simulink model "ModeStatAndRsp"  (R2018b)
settings: Solver=FixedStepDiscrete  StartTime=0.0  StopTime=10.0  FixedStep=0.01  RelTol=1e-3
undefined symbols (not defined in the file): c_RecvL, c_RecvLR, c_RecvR, IfVeSMSeStNumConfig, KeSMSbMdChime2Enable_Val, KeSMSbSRSPosNumConfig_Val, KeSMSuChmReqDurnTm_Val, KeSMSuChmReqIntlTm_Val, KeSMSuRspStatHldTm_Val, MdRspLocal1, MdTp1, ModeNum, PowerMode1, SrcReqTp1, srsconvert
libraries: RspLib x47, simulink x1
(part 5 of 8)

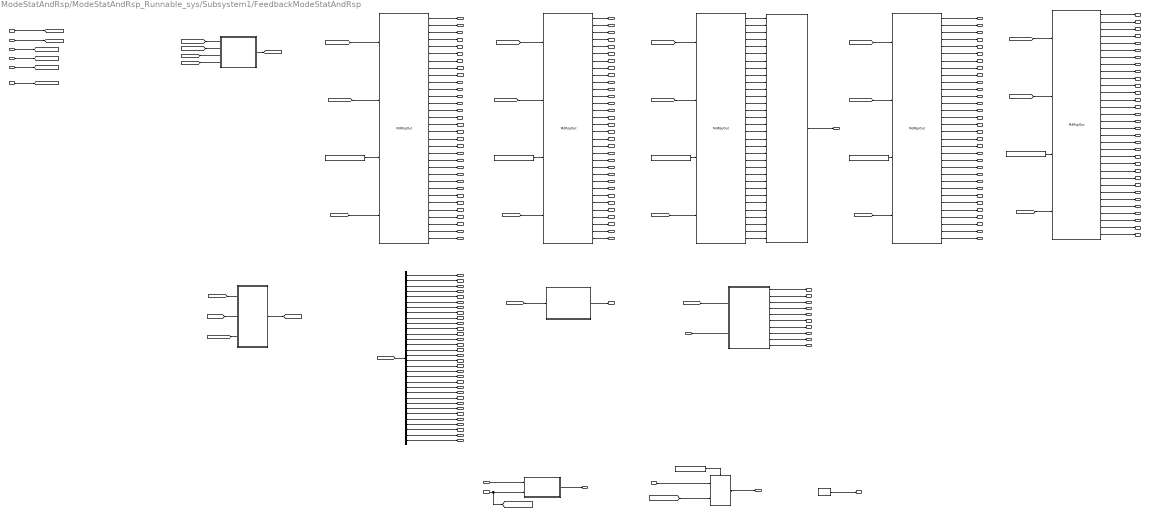
== system ModeStatAndRsp/ModeStatAndRsp_Runnable_sys/Subsystem1/FeedbackModeStatAndRsp ==
  note: REQ_MSM_479
  note: <REQ_MSM_528>
  note: <REQ_MSM_490><REQ_MSM_491>
  note: <REQ_MSM_495>
  note: <REQ_MSM_489>
  note: <REQ_MSM_492><REQ_MSM_493>
  note: <REQ_MSM_492><REQ_MSM_493>
  note: <REQ_MSM_492> <REQ_MSM_493>
  note: 0x3A6
  note: SRSLIN
  note: 0x3A7
  note: <REQ_MSM_270><REQ_MSM_ 405 > <REQ_MSM_ 416 >
  rspStateHldTm : Inport
  PwrMdChked : Inport  Port=2
  ChmMgrStat : Inport  Port=3
  ModeState32 : Inport  Port=4
  ModeStateBus : Inport  Port=5
  isArrivedAtTargetPos : Inport  Port=6
  ModeSrcTp : Inport  Port=7
  ModeRsp : Inport  Port=8
  PosArray_Val_read : Inport  Port=9
  MdExit : Inport  Port=10
  All32in1 : Subsystem
  Bus Selector : BusSelector  OutputSignals=Md1Stat,Md2Stat,Md3Stat,Md4Stat,Md5Stat,Md6Stat,Md7Stat,Md8Stat,Md9Stat,Md10Stat,Md11Stat,Md12Stat,Md13Stat,Md14Stat,Md15Stat,Md16Stat,Md17Stat,Md18Stat,Md19Stat,Md20Stat,Md21Stat,Md22Stat,Md23Stat,Md24Stat,Md25Stat,Md26Stat,Md27Stat,Md28Stat,Md29Stat,Md30Stat,Md31Stat,Md32Stat
  Chime2_3A6 : Subsystem
  Constant : Constant  Value=3  OutDataTypeStr=uint8
  Constant4 : Constant  Value=SrcReqTp1.SrcReqTp_Remote  OutDataTypeStr=Enum:SrcReqTp1
  Constant5 : Constant  Value=SrcReqTp1.SrcReqTp_HMI  OutDataTypeStr=Enum:SrcReqTp1
  Constant6 : Constant  Value=SrcReqTp1.SrcReqTp_SRS  OutDataTypeStr=Enum:SrcReqTp1
  Constant7 : Constant  Value=SrcReqTp1.SrcReqTp_HMI2L  OutDataTypeStr=Enum:SrcReqTp1
  Constant8 : Constant  Value=SrcReqTp1.SrcReqTp_HMI2R  OutDataTypeStr=Enum:SrcReqTp1
  FeedbackPassCmprtHMIDisCmd : Subsystem
  MdRspOut{1..5} (5 alike) : RspLib/MdRspOut  SystemSampleTime=-1
  MdStatComm : Subsystem
  PA_KeSMSbMdChime2Enable_Val : Constant  Value=KeSMSbMdChime2Enable_Val
  RspComm : Subsystem
  StPassCmprtMdCrtMdStat_3A6 : Subsystem
  Subsystem3 : Subsystem
  StPassCmprtMdHMIDisCmd : Outport  VectorParamsAs1DForOutWhenUnconnected=on
  IfVeSMSeStPassCmprtMdNoti2ChmEvntStat_Val_write : Outport  Port=2  VectorParamsAs1DForOutWhenUnconnected=on
  SRSCrtMdIndTyp_67_2_Val_write : Outport  Port=3  VectorParamsAs1DForOutWhenUnconnected=on
  StPassCmprtMdCrtMdStat : Outport  Port=4
  StPassCmprtMd1RclRspStat : Outport  Port=5  VectorParamsAs1DForOutWhenUnconnected=on
  StPassCmprtMd2RclRspStat : Outport  Port=6  VectorParamsAs1DForOutWhenUnconnected=on
  StPassCmprtMd3RclRspStat : Outport  Port=7  VectorParamsAs1DForOutWhenUnconnected=on
  StPassCmprtMd4RclRspStat : Outport  Port=8  VectorParamsAs1DForOutWhenUnconnected=on
  StPassCmprtMd5RclRspStat : Outport  Port=9  VectorParamsAs1DForOutWhenUnconnected=on
  StPassCmprtMd6RclRspStat : Outport  Port=10  VectorParamsAs1DForOutWhenUnconnected=on
  StPassCmprtMd7RclRspStat : Outport  Port=11  VectorParamsAs1DForOutWhenUnconnected=on
  StPassCmprtMd8RclRspStat : Outport  Port=12  VectorParamsAs1DForOutWhenUnconnected=on
  StPassCmprtMd9RclRspStat : Outport  Port=13  VectorParamsAs1DForOutWhenUnconnected=on
  StPassCmprtMd10RclRspStat : Outport  Port=14  VectorParamsAs1DForOutWhenUnconnected=on
  StPassCmprtMd11RclRspStat : Outport  Port=15  VectorParamsAs1DForOutWhenUnconnected=on
  StPassCmprtMd12RclRspStat : Outport  Port=16  VectorParamsAs1DForOutWhenUnconnected=on
  StPassCmprtMd13RclRspStat : Outport  Port=17  VectorParamsAs1DForOutWhenUnconnected=on
  StPassCmprtMd14RclRspStat : Outport  Port=18  VectorParamsAs1DForOutWhenUnconnected=on
  StPassCmprtMd15RclRspStat : Outport  Port=19  VectorParamsAs1DForOutWhenUnconnected=on
  StPassCmprtMd16RclRspStat : Outport  Port=20  VectorParamsAs1DForOutWhenUnconnected=on
  StPassCmprtMd17RclRspStat : Outport  Port=21  VectorParamsAs1DForOutWhenUnconnected=on
  StPassCmprtMd18RclRspStat : Outport  Port=22  VectorParamsAs1DForOutWhenUnconnected=on
  StPassCmprtMd19RclRspStat : Outport  Port=23  VectorParamsAs1DForOutWhenUnconnected=on
  StPassCmprtMd20RclRspStat : Outport  Port=24  VectorParamsAs1DForOutWhenUnconnected=on
  StPassCmprtMd21RclRspStat : Outport  Port=25  VectorParamsAs1DForOutWhenUnconnected=on
  StPassCmprtMd22RclRspStat : Outport  Port=26  VectorParamsAs1DForOutWhenUnconnected=on
  StPassCmprtMd23RclRspStat : Outport  Port=27  VectorParamsAs1DForOutWhenUnconnected=on
  StPassCmprtMd24RclRspStat : Outport  Port=28  VectorParamsAs1DForOutWhenUnconnected=on
  StPassCmprtMd25RclRspStat : Outport  Port=29  VectorParamsAs1DForOutWhenUnconnected=on
  StPassCmprtMd26RclRspStat : Outport  Port=30  VectorParamsAs1DForOutWhenUnconnected=on
  StPassCmprtMd27RclRspStat : Outport  Port=31  VectorParamsAs1DForOutWhenUnconnected=on
  StPassCmprtMd28RclRspStat : Outport  Port=32  VectorParamsAs1DForOutWhenUnconnected=on
  StPassCmprtMd29RclRspStat : Outport  Port=33  VectorParamsAs1DForOutWhenUnconnected=on
  StPassCmprtMd30RclRspStat : Outport  Port=34  VectorParamsAs1DForOutWhenUnconnected=on
  StPassCmprtMd31RclRspStat : Outport  Port=35  VectorParamsAs1DForOutWhenUnconnected=on
  StPassCmprtMd32RclRspStat : Outport  Port=36  VectorParamsAs1DForOutWhenUnconnected=on
  StPassCmprtMd_RfCtrl_Sw_RclRspStat : Outport  Port=37  VectorParamsAs1DForOutWhenUnconnected=on
  StSrv_StMd1_Rsp : Outport  Port=38  VectorParamsAs1DForOutWhenUnconnected=on
  StSrv_StMd2_Rsp : Outport  Port=39  VectorParamsAs1DForOutWhenUnconnected=on
  StSrv_StMd3_Rsp : Outport  Port=40  VectorParamsAs1DForOutWhenUnconnected=on
  StSrv_StMd4_Rsp : Outport  Port=41  VectorParamsAs1DForOutWhenUnconnected=on
  StSrv_StMd5_Rsp : Outport  Port=42  VectorParamsAs1DForOutWhenUnconnected=on
  StSrv_StMd6_Rsp : Outport  Port=43  VectorParamsAs1DForOutWhenUnconnected=on
  StSrv_StMd7_Rsp : Outport  Port=44  VectorParamsAs1DForOutWhenUnconnected=on
  StSrv_StMd8_Rsp : Outport  Port=45  VectorParamsAs1DForOutWhenUnconnected=on
  StSrv_StMd9_Rsp : Outport  Port=46  VectorParamsAs1DForOutWhenUnconnected=on
  StSrv_StMd10_Rsp : Outport  Port=47  VectorParamsAs1DForOutWhenUnconnected=on
  StSrv_StMd11_Rsp : Outport  Port=48  VectorParamsAs1DForOutWhenUnconnected=on
  StSrv_StMd12_Rsp : Outport  Port=49  VectorParamsAs1DForOutWhenUnconnected=on
  StSrv_StMd13_Rsp : Outport  Port=50  VectorParamsAs1DForOutWhenUnconnected=on
  StSrv_StMd14_Rsp : Outport  Port=51  VectorParamsAs1DForOutWhenUnconnected=on
  StSrv_StMd15_Rsp : Outport  Port=52  VectorParamsAs1DForOutWhenUnconnected=on
  StSrv_StMd16_Rsp : Outport  Port=53  VectorParamsAs1DForOutWhenUnconnected=on
  StSrv_StMd17_Rsp : Outport  Port=54  VectorParamsAs1DForOutWhenUnconnected=on
  StSrv_StMd18_Rsp : Outport  Port=55  VectorParamsAs1DForOutWhenUnconnected=on
  StSrv_StMd19_Rsp : Outport  Port=56  VectorParamsAs1DForOutWhenUnconnected=on
  StSrv_StMd20_Rsp : Outport  Port=57  VectorParamsAs1DForOutWhenUnconnected=on
  StSrv_StMd21_Rsp : Outport  Port=58  VectorParamsAs1DForOutWhenUnconnected=on
  StSrv_StMd22_Rsp : Outport  Port=59  VectorParamsAs1DForOutWhenUnconnected=on
  StSrv_StMd23_Rsp : Outport  Port=60  VectorParamsAs1DForOutWhenUnconnected=on
  StSrv_StMd24_Rsp : Outport  Port=61  VectorParamsAs1DForOutWhenUnconnected=on
  StSrv_StMd25_Rsp : Outport  Port=62  VectorParamsAs1DForOutWhenUnconnected=on
  StSrv_StMd26_Rsp : Outport  Port=63  VectorParamsAs1DForOutWhenUnconnected=on
  StSrv_StMd27_Rsp : Outport  Port=64  VectorParamsAs1DForOutWhenUnconnected=on
  StSrv_StMd28_Rsp : Outport  Port=65  VectorParamsAs1DForOutWhenUnconnected=on
  StSrv_StMd29_Rsp : Outport  Port=66  VectorParamsAs1DForOutWhenUnconnected=on
  StSrv_StMd30_Rsp : Outport  Port=67  VectorParamsAs1DForOutWhenUnconnected=on
  StSrv_StMd31_Rsp : Outport  Port=68  VectorParamsAs1DForOutWhenUnconnected=on
  StSrv_StMd32_Rsp : Outport  Port=69  VectorParamsAs1DForOutWhenUnconnected=on
  HMI_2L_StMd1_Rsp : Outport  Port=70  VectorParamsAs1DForOutWhenUnconnected=on
  HMI_2L_StMd2_Rsp : Outport  Port=71  VectorParamsAs1DForOutWhenUnconnected=on
  HMI_2L_StMd3_Rsp : Outport  Port=72  VectorParamsAs1DForOutWhenUnconnected=on
  HMI_2L_StMd4_Rsp : Outport  Port=73  VectorParamsAs1DForOutWhenUnconnected=on
  HMI_2L_StMd5_Rsp : Outport  Port=74  VectorParamsAs1DForOutWhenUnconnected=on
  HMI_2L_StMd6_Rsp : Outport  Port=75  VectorParamsAs1DForOutWhenUnconnected=on
  HMI_2L_StMd7_Rsp : Outport  Port=76  VectorParamsAs1DForOutWhenUnconnected=on
  HMI_2L_StMd8_Rsp : Outport  Port=77  VectorParamsAs1DForOutWhenUnconnected=on
  HMI_2L_StMd9_Rsp : Outport  Port=78  VectorParamsAs1DForOutWhenUnconnected=on
  HMI_2L_StMd10_Rsp : Outport  Port=79  VectorParamsAs1DForOutWhenUnconnected=on
  HMI_2L_StMd11_Rsp : Outport  Port=80  VectorParamsAs1DForOutWhenUnconnected=on
  HMI_2L_StMd12_Rsp : Outport  Port=81  VectorParamsAs1DForOutWhenUnconnected=on
  HMI_2L_StMd13_Rsp : Outport  Port=82  VectorParamsAs1DForOutWhenUnconnected=on
  HMI_2L_StMd14_Rsp : Outport  Port=83  VectorParamsAs1DForOutWhenUnconnected=on
  HMI_2L_StMd15_Rsp : Outport  Port=84  VectorParamsAs1DForOutWhenUnconnected=on
  HMI_2L_StMd16_Rsp : Outport  Port=85  VectorParamsAs1DForOutWhenUnconnected=on
  HMI_2L_StMd17_Rsp : Outport  Port=86  VectorParamsAs1DForOutWhenUnconnected=on
  HMI_2L_StMd18_Rsp : Outport  Port=87  VectorParamsAs1DForOutWhenUnconnected=on
  HMI_2L_StMd19_Rsp : Outport  Port=88  VectorParamsAs1DForOutWhenUnconnected=on
  HMI_2L_StMd20_Rsp : Outport  Port=89  VectorParamsAs1DForOutWhenUnconnected=on
  HMI_2L_StMd21_Rsp : Outport  Port=90  VectorParamsAs1DForOutWhenUnconnected=on
  HMI_2L_StMd22_Rsp : Outport  Port=91  VectorParamsAs1DForOutWhenUnconnected=on
  HMI_2L_StMd23_Rsp : Outport  Port=92  VectorParamsAs1DForOutWhenUnconnected=on
  HMI_2L_StMd24_Rsp : Outport  Port=93  VectorParamsAs1DForOutWhenUnconnected=on
  HMI_2L_StMd25_Rsp : Outport  Port=94  VectorParamsAs1DForOutWhenUnconnected=on
  HMI_2L_StMd26_Rsp : Outport  Port=95  VectorParamsAs1DForOutWhenUnconnected=on
  HMI_2L_StMd27_Rsp : Outport  Port=96  VectorParamsAs1DForOutWhenUnconnected=on
  HMI_2L_StMd28_Rsp : Outport  Port=97  VectorParamsAs1DForOutWhenUnconnected=on
  HMI_2L_StMd29_Rsp : Outport  Port=98  VectorParamsAs1DForOutWhenUnconnected=on
  HMI_2L_StMd30_Rsp : Outport  Port=99  VectorParamsAs1DForOutWhenUnconnected=on
  HMI_2L_StMd31_Rsp : Outport  Port=100  VectorParamsAs1DForOutWhenUnconnected=on
  HMI_2L_StMd32_Rsp : Outport  Port=101  VectorParamsAs1DForOutWhenUnconnected=on
  HMI_2R_StMd1_Rsp : Outport  Port=102  VectorParamsAs1DForOutWhenUnconnected=on
  HMI_2R_StMd2_Rsp : Outport  Port=103  VectorParamsAs1DForOutWhenUnconnected=on
  HMI_2R_StMd3_Rsp : Outport  Port=104  VectorParamsAs1DForOutWhenUnconnected=on
  HMI_2R_StMd4_Rsp : Outport  Port=105  VectorParamsAs1DForOutWhenUnconnected=on
  HMI_2R_StMd5_Rsp : Outport  Port=106  VectorParamsAs1DForOutWhenUnconnected=on
  HMI_2R_StMd6_Rsp : Outport  Port=107  VectorParamsAs1DForOutWhenUnconnected=on
  HMI_2R_StMd7_Rsp : Outport  Port=108  VectorParamsAs1DForOutWhenUnconnected=on
  HMI_2R_StMd8_Rsp : Outport  Port=109  VectorParamsAs1DForOutWhenUnconnected=on
  HMI_2R_StMd9_Rsp : Outport  Port=110  VectorParamsAs1DForOutWhenUnconnected=on
  HMI_2R_StMd10_Rsp : Outport  Port=111  VectorParamsAs1DForOutWhenUnconnected=on
  HMI_2R_StMd11_Rsp : Outport  Port=112  VectorParamsAs1DForOutWhenUnconnected=on
  HMI_2R_StMd12_Rsp : Outport  Port=113  VectorParamsAs1DForOutWhenUnconnected=on
  HMI_2R_StMd13_Rsp : Outport  Port=114  VectorParamsAs1DForOutWhenUnconnected=on
  HMI_2R_StMd14_Rsp : Outport  Port=115  VectorParamsAs1DForOutWhenUnconnected=on
  HMI_2R_StMd15_Rsp : Outport  Port=116  VectorParamsAs1DForOutWhenUnconnected=on
  HMI_2R_StMd16_Rsp : Outport  Port=117  VectorParamsAs1DForOutWhenUnconnected=on
  HMI_2R_StMd17_Rsp : Outport  Port=118  VectorParamsAs1DForOutWhenUnconnected=on
  HMI_2R_StMd18_Rsp : Outport  Port=119  VectorParamsAs1DForOutWhenUnconnected=on
  HMI_2R_StMd19_Rsp : Outport  Port=120  VectorParamsAs1DForOutWhenUnconnected=on
  HMI_2R_StMd20_Rsp : Outport  Port=121  VectorParamsAs1DForOutWhenUnconnected=on
  HMI_2R_StMd21_Rsp : Outport  Port=122  VectorParamsAs1DForOutWhenUnconnected=on
  HMI_2R_StMd22_Rsp : Outport  Port=123  VectorParamsAs1DForOutWhenUnconnected=on
  HMI_2R_StMd23_Rsp : Outport  Port=124  VectorParamsAs1DForOutWhenUnconnected=on
  HMI_2R_StMd24_Rsp : Outport  Port=125  VectorParamsAs1DForOutWhenUnconnected=on
  HMI_2R_StMd25_Rsp : Outport  Port=126  VectorParamsAs1DForOutWhenUnconnected=on
  HMI_2R_StMd26_Rsp : Outport  Port=127  VectorParamsAs1DForOutWhenUnconnected=on
  HMI_2R_StMd27_Rsp : Outport  Port=128  VectorParamsAs1DForOutWhenUnconnected=on
  HMI_2R_StMd28_Rsp : Outport  Port=129  VectorParamsAs1DForOutWhenUnconnected=on
  HMI_2R_StMd29_Rsp : Outport  Port=130  VectorParamsAs1DForOutWhenUnconnected=on
  HMI_2R_StMd30_Rsp : Outport  Port=131  VectorParamsAs1DForOutWhenUnconnected=on
  HMI_2R_StMd31_Rsp : Outport  Port=132  VectorParamsAs1DForOutWhenUnconnected=on
  HMI_2R_StMd32_Rsp : Outport  Port=133  VectorParamsAs1DForOutWhenUnconnected=on
  StPassCmprtMd_Md1_CrtStat : Outport  Port=134
  StPassCmprtMd_Md2_CrtStat : Outport  Port=135
  StPassCmprtMd_Md3_CrtStat : Outport  Port=136
  StPassCmprtMd_Md4_CrtStat : Outport  Port=137
  StPassCmprtMd_Md5_CrtStat : Outport  Port=138
  StPassCmprtMd_Md6_CrtStat : Outport  Port=139
  StPassCmprtMd_Md7_CrtStat : Outport  Port=140
  StPassCmprtMd_Md8_CrtStat : Outport  Port=141
  StPassCmprtMd_Md9_CrtStat : Outport  Port=142
  StPassCmprtMd_Md10_CrtStat : Outport  Port=143
  StPassCmprtMd_Md11_CrtStat : Outport  Port=144
  StPassCmprtMd_Md12_CrtStat : Outport  Port=145
  StPassCmprtMd_Md13_CrtStat : Outport  Port=146
  StPassCmprtMd_Md14_CrtStat : Outport  Port=147
  StPassCmprtMd_Md15_CrtStat : Outport  Port=148
  StPassCmprtMd_Md16_CrtStat : Outport  Port=149
  StPassCmprtMd_Md17_CrtStat : Outport  Port=150
  StPassCmprtMd_Md18_CrtStat : Outport  Port=151
  StPassCmprtMd_Md19_CrtStat : Outport  Port=152
  StPassCmprtMd_Md20_CrtStat : Outport  Port=153
  StPassCmprtMd_Md21_CrtStat : Outport  Port=154
  StPassCmprtMd_Md22_CrtStat : Outport  Port=155
  StPassCmprtMd_Md23_CrtStat : Outport  Port=156
  StPassCmprtMd_Md24_CrtStat : Outport  Port=157
  StPassCmprtMd_Md25_CrtStat : Outport  Port=158
  StPassCmprtMd_Md26_CrtStat : Outport  Port=159
  StPassCmprtMd_Md27_CrtStat : Outport  Port=160
  StPassCmprtMd_Md28_CrtStat : Outport  Port=161
  StPassCmprtMd_Md29_CrtStat : Outport  Port=162
  StPassCmprtMd_Md30_CrtStat : Outport  Port=163
  StPassCmprtMd_Md31_CrtStat : Outport  Port=164
  StPassCmprtMd_Md32_CrtStat : Outport  Port=165
  SRSCrt_MdSw1_Stat_67_2 : Outport  Port=166
  SRSCrt_MdSw2_Stat_67_2 : Outport  Port=167
  SRSCrt_MdSw3_Stat_67_2 : Outport  Port=168
  SRSCrt_MdSw4_Stat_67_2 : Outport  Port=169
  SRSCrt_MdSw5_Stat_67_2 : Outport  Port=170
  SRSCrt_MdSw6_Stat_67_2 : Outport  Port=171
  SRSCrt_MdSw7_Stat_67_2 : Outport  Port=172
  SRSCrt_MdSw8_Stat_67_2 : Outport  Port=173
  SRSCrt_MdSw9_Stat_67_2 : Outport  Port=174
  SRSCrt_MdSw10_Stat_67_2 : Outport  Port=175
  wires:
  rspStateHldTm/1 -> [rspStateHldTm]
  MdRspOut5/1 -> StPassCmprtMd1RclRspStat/1
  StPassCmprtMdCrtMdStat_3A6/1(StPassCmprtMdCrtMdStat) -> StPassCmprtMdCrtMdStat/1
  FeedbackPassCmprtHMIDisCmd/1(StPassCmprtMdHMIDisCmd) -> StPassCmprtMdHMIDisCmd/1
  PwrMdChked/1 -> FeedbackPassCmprtHMIDisCmd/1(powerMode)
  MdRspOut2/6 -> StSrv_StMd6_Rsp/1
  MdRspOut2/7 -> StSrv_StMd7_Rsp/1
  MdRspOut2/8 -> StSrv_StMd8_Rsp/1
  MdRspOut2/4 -> StSrv_StMd4_Rsp/1
  MdRspOut2/5 -> StSrv_StMd5_Rsp/1
  MdRspOut2/1 -> StSrv_StMd1_Rsp/1
  MdRspOut2/2 -> StSrv_StMd2_Rsp/1
  MdRspOut2/3 -> StSrv_StMd3_Rsp/1
  Constant4/1 -> MdRspOut2/3
  Chime2_3A6/1(Out1) -> IfVeSMSeStPassCmprtMdNoti2ChmEvntStat_Val_write/1
  ChmMgrStat/1 -> Chime2_3A6/1(ChmMgrStat)
  Constant/1 -> SRSCrtMdIndTyp_67_2_Val_write/1
  ModeSrcTp/1 -> [ModeSrcTp]
  ModeRsp/1 -> [ModeRsp]
  ModeStateBus/1 -> [ModeStateBus]
  [MdRsp] -> MdRspOut2/1
  [ModeSrcTp] -> MdRspOut2/2
  [ModeSrcTp] -> MdRspOut5/2
  [MdRsp] -> MdRspOut5/1
  ModeState32/1 -> [ModeState32], FeedbackPassCmprtHMIDisCmd/2(ModeState32)
  [ModeState32] -> Chime2_3A6/2(ModeState32)
  [ModeStateBus] -> RspComm/1(oModeStateBus)
  [ModeRsp] -> RspComm/2(oModeRsp)
  [rspStateHldTm] -> RspComm/3(rspStateHldTm)
  RspComm/1(Rsp) -> [MdRsp]
  MdRspOut5/3 -> StPassCmprtMd3RclRspStat/1
  MdRspOut5/4 -> StPassCmprtMd4RclRspStat/1
  MdRspOut5/2 -> StPassCmprtMd2RclRspStat/1
  MdRspOut5/5 -> StPassCmprtMd5RclRspStat/1
  MdRspOut5/6 -> StPassCmprtMd6RclRspStat/1
  MdRspOut5/7 -> StPassCmprtMd7RclRspStat/1
  MdRspOut5/8 -> StPassCmprtMd8RclRspStat/1
  MdRspOut5/9 -> StPassCmprtMd9RclRspStat/1
  MdRspOut5/10 -> StPassCmprtMd10RclRspStat/1
  MdRspOut5/11 -> StPassCmprtMd11RclRspStat/1
  MdRspOut5/12 -> StPassCmprtMd12RclRspStat/1
  MdRspOut5/13 -> StPassCmprtMd13RclRspStat/1
  MdRspOut5/14 -> StPassCmprtMd14RclRspStat/1
  MdRspOut5/15 -> StPassCmprtMd15RclRspStat/1
  MdRspOut5/16 -> StPassCmprtMd16RclRspStat/1
  MdRspOut5/17 -> StPassCmprtMd17RclRspStat/1
  MdRspOut5/18 -> StPassCmprtMd18RclRspStat/1
  MdRspOut5/19 -> StPassCmprtMd19RclRspStat/1
  MdRspOut5/20 -> StPassCmprtMd20RclRspStat/1
  MdRspOut5/21 -> StPassCmprtMd21RclRspStat/1
  MdRspOut5/22 -> StPassCmprtMd22RclRspStat/1
  MdRspOut5/23 -> StPassCmprtMd23RclRspStat/1
  MdRspOut5/24 -> StPassCmprtMd24RclRspStat/1
  MdRspOut5/25 -> StPassCmprtMd25RclRspStat/1
  MdRspOut5/26 -> StPassCmprtMd26RclRspStat/1
  MdRspOut5/27 -> StPassCmprtMd27RclRspStat/1
  MdRspOut5/28 -> StPassCmprtMd28RclRspStat/1
  MdRspOut5/29 -> StPassCmprtMd29RclRspStat/1
  MdRspOut5/30 -> StPassCmprtMd30RclRspStat/1
  MdRspOut5/31 -> StPassCmprtMd31RclRspStat/1
  MdRspOut5/32 -> StPassCmprtMd32RclRspStat/1
  Constant5/1 -> MdRspOut5/3
  isArrivedAtTargetPos/1 -> [isArrivedAtTargetPos]
  [isArrivedAtTargetPos] -> RspComm/4(IsArrivedAtTrgtPos)
  [MdRsp] -> MdRspOut1/1
  [ModeSrcTp] -> MdRspOut1/2
  Constant6/1 -> MdRspOut1/3
  All32in1/1(Allin1Rsp) -> StPassCmprtMd_RfCtrl_Sw_RclRspStat/1
  MdRspOut1/1 -> All32in1/1(Md1Rsp)
  MdRspOut1/2 -> All32in1/2(Md2Rsp)
  MdRspOut1/3 -> All32in1/3(Md3Rsp)
  MdRspOut1/4 -> All32in1/4(Md4Rsp)
  MdRspOut1/5 -> All32in1/5(Md5Rsp)
  MdRspOut1/6 -> All32in1/6(Md6Rsp)
  MdRspOut1/7 -> All32in1/7(Md7Rsp)
  MdRspOut1/8 -> All32in1/8(Md8Rsp)
  MdRspOut1/9 -> All32in1/9(Md9Rsp)
  MdRspOut1/10 -> All32in1/10(Md10Rsp)
  MdRspOut1/11 -> All32in1/11(Md11Rsp)
  MdRspOut1/12 -> All32in1/12(Md12Rsp)
  MdRspOut1/13 -> All32in1/13(Md13Rsp)
  MdRspOut1/14 -> All32in1/14(Md14Rsp)
  MdRspOut1/15 -> All32in1/15(Md15Rsp)
  MdRspOut1/16 -> All32in1/16(Md16Rsp)
  MdRspOut1/17 -> All32in1/17(Md17Rsp)
  MdRspOut1/18 -> All32in1/18(Md18Rsp)
  MdRspOut1/19 -> All32in1/19(Md19Rsp)
  MdRspOut1/20 -> All32in1/20(Md20Rsp)
  MdRspOut1/21 -> All32in1/21(Md21Rsp)
  MdRspOut1/22 -> All32in1/22(Md22Rsp)
  MdRspOut1/23 -> All32in1/23(Md23Rsp)
  MdRspOut1/24 -> All32in1/24(Md24Rsp)
  MdRspOut1/25 -> All32in1/25(Md25Rsp)
  MdRspOut1/26 -> All32in1/26(Md26Rsp)
  MdRspOut1/27 -> All32in1/27(Md27Rsp)
  MdRspOut1/28 -> All32in1/28(Md28Rsp)
  MdRspOut1/29 -> All32in1/29(Md29Rsp)
  MdRspOut1/30 -> All32in1/30(Md30Rsp)
  MdRspOut1/31 -> All32in1/31(Md31Rsp)
  MdRspOut1/32 -> All32in1/32(Md32Rsp)
  MdRspOut2/9 -> StSrv_StMd9_Rsp/1
  MdRspOut2/10 -> StSrv_StMd10_Rsp/1
  MdRspOut2/11 -> StSrv_StMd11_Rsp/1
  MdRspOut2/12 -> StSrv_StMd12_Rsp/1
  MdRspOut2/13 -> StSrv_StMd13_Rsp/1
  MdRspOut2/14 -> StSrv_StMd14_Rsp/1
  MdRspOut2/15 -> StSrv_StMd15_Rsp/1
  MdRspOut2/16 -> StSrv_StMd16_Rsp/1
  MdRspOut2/17 -> StSrv_StMd17_Rsp/1
  MdRspOut2/18 -> StSrv_StMd18_Rsp/1
  MdRspOut2/19 -> StSrv_StMd19_Rsp/1
  MdRspOut2/20 -> StSrv_StMd20_Rsp/1
  MdRspOut2/21 -> StSrv_StMd21_Rsp/1
  MdRspOut2/22 -> StSrv_StMd22_Rsp/1
  MdRspOut2/23 -> StSrv_StMd23_Rsp/1
  MdRspOut2/24 -> StSrv_StMd24_Rsp/1
  MdRspOut2/25 -> StSrv_StMd25_Rsp/1
  MdRspOut2/26 -> StSrv_StMd26_Rsp/1
  MdRspOut2/27 -> StSrv_StMd27_Rsp/1
  MdRspOut2/28 -> StSrv_StMd28_Rsp/1
  MdRspOut2/29 -> StSrv_StMd29_Rsp/1
  MdRspOut2/30 -> StSrv_StMd30_Rsp/1
  MdRspOut2/31 -> StSrv_StMd31_Rsp/1
  MdRspOut2/32 -> StSrv_StMd32_Rsp/1
  [MdRsp] -> MdRspOut3/1
  [ModeSrcTp] -> MdRspOut3/2
  Constant7/1 -> MdRspOut3/3
  [ModeSrcTp] -> MdRspOut4/2
  [MdRsp] -> MdRspOut4/1
  Constant8/1 -> MdRspOut4/3
  MdRspOut3/1 -> HMI_2L_StMd1_Rsp/1
  MdRspOut3/2 -> HMI_2L_StMd2_Rsp/1
  MdRspOut3/3 -> HMI_2L_StMd3_Rsp/1
  MdRspOut3/4 -> HMI_2L_StMd4_Rsp/1
  MdRspOut3/5 -> HMI_2L_StMd5_Rsp/1
  MdRspOut3/6 -> HMI_2L_StMd6_Rsp/1
  MdRspOut3/7 -> HMI_2L_StMd7_Rsp/1
  MdRspOut3/8 -> HMI_2L_StMd8_Rsp/1
  MdRspOut3/9 -> HMI_2L_StMd9_Rsp/1
  MdRspOut3/10 -> HMI_2L_StMd10_Rsp/1
  MdRspOut3/11 -> HMI_2L_StMd11_Rsp/1
  MdRspOut3/12 -> HMI_2L_StMd12_Rsp/1
  MdRspOut3/13 -> HMI_2L_StMd13_Rsp/1
  MdRspOut3/14 -> HMI_2L_StMd14_Rsp/1
  MdRspOut3/15 -> HMI_2L_StMd15_Rsp/1
  MdRspOut3/16 -> HMI_2L_StMd16_Rsp/1
  MdRspOut3/17 -> HMI_2L_StMd17_Rsp/1
  MdRspOut3/18 -> HMI_2L_StMd18_Rsp/1
  MdRspOut3/19 -> HMI_2L_StMd19_Rsp/1
  MdRspOut3/20 -> HMI_2L_StMd20_Rsp/1
  MdRspOut3/21 -> HMI_2L_StMd21_Rsp/1
  MdRspOut3/22 -> HMI_2L_StMd22_Rsp/1
  MdRspOut3/23 -> HMI_2L_StMd23_Rsp/1
  MdRspOut3/24 -> HMI_2L_StMd24_Rsp/1
  MdRspOut3/25 -> HMI_2L_StMd25_Rsp/1
  MdRspOut3/26 -> HMI_2L_StMd26_Rsp/1
  MdRspOut3/27 -> HMI_2L_StMd27_Rsp/1
  MdRspOut3/28 -> HMI_2L_StMd28_Rsp/1
  MdRspOut3/29 -> HMI_2L_StMd29_Rsp/1
  MdRspOut3/30 -> HMI_2L_StMd30_Rsp/1
  MdRspOut3/31 -> HMI_2L_StMd31_Rsp/1
  MdRspOut3/32 -> HMI_2L_StMd32_Rsp/1
  MdRspOut4/1 -> HMI_2R_StMd1_Rsp/1
  MdRspOut4/31 -> HMI_2R_StMd31_Rsp/1
  MdRspOut4/29 -> HMI_2R_StMd29_Rsp/1
  MdRspOut4/28 -> HMI_2R_StMd28_Rsp/1
  MdRspOut4/26 -> HMI_2R_StMd26_Rsp/1
  MdRspOut4/32 -> HMI_2R_StMd32_Rsp/1
  MdRspOut4/27 -> HMI_2R_StMd27_Rsp/1
  MdRspOut4/23 -> HMI_2R_StMd23_Rsp/1
  MdRspOut4/24 -> HMI_2R_StMd24_Rsp/1
  MdRspOut4/22 -> HMI_2R_StMd22_Rsp/1
  MdRspOut4/19 -> HMI_2R_StMd19_Rsp/1
  MdRspOut4/20 -> HMI_2R_StMd20_Rsp/1
  MdRspOut4/18 -> HMI_2R_StMd18_Rsp/1
  MdRspOut4/16 -> HMI_2R_StMd16_Rsp/1
  MdRspOut4/17 -> HMI_2R_StMd17_Rsp/1
  MdRspOut4/15 -> HMI_2R_StMd15_Rsp/1
  MdRspOut4/12 -> HMI_2R_StMd12_Rsp/1
  MdRspOut4/11 -> HMI_2R_StMd11_Rsp/1
  MdRspOut4/10 -> HMI_2R_StMd10_Rsp/1
  MdRspOut4/5 -> HMI_2R_StMd5_Rsp/1
  MdRspOut4/7 -> HMI_2R_StMd7_Rsp/1
  MdRspOut4/30 -> HMI_2R_StMd30_Rsp/1
  MdRspOut4/8 -> HMI_2R_StMd8_Rsp/1
  MdRspOut4/21 -> HMI_2R_StMd21_Rsp/1
  MdRspOut4/6 -> HMI_2R_StMd6_Rsp/1
  MdRspOut4/4 -> HMI_2R_StMd4_Rsp/1
  MdRspOut4/25 -> HMI_2R_StMd25_Rsp/1
  MdRspOut4/3 -> HMI_2R_StMd3_Rsp/1
  MdRspOut4/13 -> HMI_2R_StMd13_Rsp/1
  MdRspOut4/2 -> HMI_2R_StMd2_Rsp/1
  MdRspOut4/9 -> HMI_2R_StMd9_Rsp/1
  MdRspOut4/14 -> HMI_2R_StMd14_Rsp/1
  [isArrivedAtTargetPos] -> MdStatComm/1(IsArrivedAtTrgtPos)
  [MdRsp] -> MdStatComm/2(Rsp)
  MdStatComm/1(MdStat) -> [MdStat]
  [MdStat] -> Bus Selector/1
  Bus Selector/1 -> StPassCmprtMd_Md1_CrtStat/1  "<Md1Stat>"
  Bus Selector/2 -> StPassCmprtMd_Md2_CrtStat/1  "<Md2Stat>"
  Bus Selector/3 -> StPassCmprtMd_Md3_CrtStat/1  "<Md3Stat>"
  Bus Selector/4 -> StPassCmprtMd_Md4_CrtStat/1  "<Md4Stat>"
  Bus Selector/5 -> StPassCmprtMd_Md5_CrtStat/1  "<Md5Stat>"
  Bus Selector/6 -> StPassCmprtMd_Md6_CrtStat/1  "<Md6Stat>"
  Bus Selector/7 -> StPassCmprtMd_Md7_CrtStat/1  "<Md7Stat>"
  Bus Selector/8 -> StPassCmprtMd_Md8_CrtStat/1  "<Md8Stat>"
  Bus Selector/9 -> StPassCmprtMd_Md9_CrtStat/1  "<Md9Stat>"
  Bus Selector/10 -> StPassCmprtMd_Md10_CrtStat/1  "<Md10Stat>"
  Bus Selector/11 -> StPassCmprtMd_Md11_CrtStat/1  "<Md11Stat>"
  Bus Selector/12 -> StPassCmprtMd_Md12_CrtStat/1  "<Md12Stat>"
  Bus Selector/13 -> StPassCmprtMd_Md13_CrtStat/1  "<Md13Stat>"
  Bus Selector/14 -> StPassCmprtMd_Md14_CrtStat/1  "<Md14Stat>"
  Bus Selector/15 -> StPassCmprtMd_Md15_CrtStat/1  "<Md15Stat>"
  Bus Selector/16 -> StPassCmprtMd_Md16_CrtStat/1  "<Md16Stat>"
  Bus Selector/17 -> StPassCmprtMd_Md17_CrtStat/1  "<Md17Stat>"
  Bus Selector/18 -> StPassCmprtMd_Md18_CrtStat/1  "<Md18Stat>"
  Bus Selector/19 -> StPassCmprtMd_Md19_CrtStat/1  "<Md19Stat>"
  Bus Selector/20 -> StPassCmprtMd_Md20_CrtStat/1  "<Md20Stat>"
  Bus Selector/21 -> StPassCmprtMd_Md21_CrtStat/1  "<Md21Stat>"
  Bus Selector/22 -> StPassCmprtMd_Md22_CrtStat/1  "<Md22Stat>"
  Bus Selector/23 -> StPassCmprtMd_Md23_CrtStat/1  "<Md23Stat>"
  Bus Selector/24 -> StPassCmprtMd_Md24_CrtStat/1  "<Md24Stat>"
  Bus Selector/25 -> StPassCmprtMd_Md25_CrtStat/1  "<Md25Stat>"
  Bus Selector/26 -> StPassCmprtMd_Md26_CrtStat/1  "<Md26Stat>"
  Bus Selector/27 -> StPassCmprtMd_Md27_CrtStat/1  "<Md27Stat>"
  Bus Selector/28 -> StPassCmprtMd_Md28_CrtStat/1  "<Md28Stat>"
  Bus Selector/29 -> StPassCmprtMd_Md29_CrtStat/1  "<Md29Stat>"
  Bus Selector/30 -> StPassCmprtMd_Md30_CrtStat/1  "<Md30Stat>"
  Bus Selector/31 -> StPassCmprtMd_Md31_CrtStat/1  "<Md31Stat>"
  Bus Selector/32 -> StPassCmprtMd_Md32_CrtStat/1  "<Md32Stat>"
  [MdStat] -> StPassCmprtMdCrtMdStat_3A6/1(MdStat)
  Subsystem3/9(SRSCrt_MdSw9_Stat_67_2) -> SRSCrt_MdSw9_Stat_67_2/1
  Subsystem3/5(SRSCrt_MdSw5_Stat_67_2) -> SRSCrt_MdSw5_Stat_67_2/1
  Subsystem3/6(SRSCrt_MdSw6_Stat_67_2) -> SRSCrt_MdSw6_Stat_67_2/1
  Subsystem3/7(SRSCrt_MdSw7_Stat_67_2) -> SRSCrt_MdSw7_Stat_67_2/1
  Subsystem3/8(SRSCrt_MdSw8_Stat_67_2) -> SRSCrt_MdSw8_Stat_67_2/1
  Subsystem3/3(SRSCrt_MdSw3_Stat_67_2) -> SRSCrt_MdSw3_Stat_67_2/1
  Subsystem3/4(SRSCrt_MdSw4_Stat_67_2) -> SRSCrt_MdSw4_Stat_67_2/1
  Subsystem3/10(SRSCrt_MdSw10_Stat_67_2) -> SRSCrt_MdSw10_Stat_67_2/1
  Subsystem3/1(SRSCrt_MdSw1_Stat_67_2) -> SRSCrt_MdSw1_Stat_67_2/1
  Subsystem3/2(SRSCrt_MdSw2_Stat_67_2) -> SRSCrt_MdSw2_Stat_67_2/1
  [MdStat] -> Subsystem3/1(MdStat)
  PosArray_Val_read/1 -> Subsystem3/2(PosArray_Val_read)
  [rspStateHldTm] -> MdRspOut2/4
  [rspStateHldTm] -> MdRspOut5/4
  [rspStateHldTm] -> MdRspOut1/4
  [rspStateHldTm] -> MdRspOut3/4
  [rspStateHldTm] -> MdRspOut4/4
  MdExit/1 -> [MdExit]
  [MdExit] -> MdStatComm/3(MdExit)
  PA_KeSMSbMdChime2Enable_Val/1 -> Chime2_3A6/Enable

== system ModeStatAndRsp/ModeStatAndRsp_Runnable_sys/Subsystem1/SRSModeCheck ==
  MdStatusBus : Inport
  MdSrcTp : Inport  Port=2
  Bus Selector2 : BusSelector  OutputSignals=Md1_En,Md2_En,Md3_En,Md4_En,Md5_En,Md6_En,Md7_En,Md8_En,Md9_En,Md10_En,Md11_En,Md12_En,Md13_En,Md14_En,Md15_En,Md16_En,Md17_En,Md18_En,Md19_En,Md20_En
  Bus Selector3 : BusSelector  OutputSignals=Md1SrcTp,Md2SrcTp,Md3SrcTp,Md4SrcTp,Md5SrcTp,Md6SrcTp,Md7SrcTp,Md8SrcTp,Md9SrcTp,Md10SrcTp,Md11SrcTp,Md12SrcTp,Md13SrcTp,Md14SrcTp,Md15SrcTp,Md16SrcTp,Md17SrcTp,Md18SrcTp,Md19SrcTp,Md20SrcTp
  Chart : Stateflow chart  TreatAsAtomicUnit=on
  Constant : Constant  Value=ModeNum  OutDataTypeStr=uint8
  Constant1 : Constant  Value=srsconvert  OutDataTypeStr=uint8
  Data Type Conversion : DataTypeConversion  OutDataTypeStr=Enum:SRSCurMode1
  Index Vector : MultiPortSwitch  DataPortOrder=Zero-based contiguous  Inputs=1  zeroidx=on
  Mux : Mux  Inputs=20
  Mux1 : Mux  Inputs=20
  SRSModeState : Outport
  wires:
  MdStatusBus/1 -> Bus Selector2/1
  MdSrcTp/1 -> Bus Selector3/1
  Bus Selector2/3 -> Mux/3  "<Md3_En>"
  Bus Selector2/2 -> Mux/2  "<Md2_En>"
  Bus Selector2/4 -> Mux/4  "<Md4_En>"
  Bus Selector2/1 -> Mux/1  "<Md1_En>"
  Bus Selector2/5 -> Mux/5  "<Md5_En>"
  Bus Selector2/6 -> Mux/6  "<Md6_En>"
  Bus Selector2/7 -> Mux/7  "<Md7_En>"
  Bus Selector2/8 -> Mux/8  "<Md8_En>"
  Bus Selector2/9 -> Mux/9  "<Md9_En>"
  Bus Selector2/10 -> Mux/10  "<Md10_En>"
  Bus Selector2/11 -> Mux/11  "<Md11_En>"
  Bus Selector2/12 -> Mux/12  "<Md12_En>"
  Bus Selector2/13 -> Mux/13  "<Md13_En>"
  Bus Selector2/14 -> Mux/14  "<Md14_En>"
  Bus Selector2/15 -> Mux/15  "<Md15_En>"
  Bus Selector3/1 -> Mux1/1  "<Md1SrcTp>"
  Bus Selector3/2 -> Mux1/2  "<Md2SrcTp>"
  Bus Selector3/3 -> Mux1/3  "<Md3SrcTp>"
  Bus Selector3/4 -> Mux1/4  "<Md4SrcTp>"
  Bus Selector3/5 -> Mux1/5  "<Md5SrcTp>"
  Bus Selector3/6 -> Mux1/6  "<Md6SrcTp>"
  Bus Selector3/7 -> Mux1/7  "<Md7SrcTp>"
  Bus Selector3/8 -> Mux1/8  "<Md8SrcTp>"
  Bus Selector3/9 -> Mux1/9  "<Md9SrcTp>"
  Bus Selector3/10 -> Mux1/10  "<Md10SrcTp>"
  Bus Selector3/11 -> Mux1/11  "<Md11SrcTp>"
  Bus Selector3/12 -> Mux1/12  "<Md12SrcTp>"
  Bus Selector3/13 -> Mux1/13  "<Md13SrcTp>"
  Bus Selector3/14 -> Mux1/14  "<Md14SrcTp>"
  Bus Selector3/15 -> Mux1/15  "<Md15SrcTp>"
  Mux/1 -> Chart/1(Md_En)
  Mux1/1 -> Chart/2(MdSrcTp)
  Constant/1 -> Chart/3(ModeNum)
  Data Type Conversion/1 -> SRSModeState/1
  Index Vector/1 -> Data Type Conversion/1
  Chart/1(U8SRSMode) -> Index Vector/1
  Constant1/1 -> Index Vector/2
  Bus Selector2/16 -> Mux/16  "<Md16_En>"
  Bus Selector2/17 -> Mux/17  "<Md17_En>"
  Bus Selector2/18 -> Mux/18  "<Md18_En>"
  Bus Selector2/19 -> Mux/19  "<Md19_En>"
  Bus Selector2/20 -> Mux/20  "<Md20_En>"
  Bus Selector3/16 -> Mux1/16  "<Md16SrcTp>"
  Bus Selector3/17 -> Mux1/17  "<Md17SrcTp>"
  Bus Selector3/18 -> Mux1/18  "<Md18SrcTp>"
  Bus Selector3/19 -> Mux1/19  "<Md19SrcTp>"
  Bus Selector3/20 -> Mux1/20  "<Md20SrcTp>"
